simulink model "HANcoder_E407_GTSync_v4"  (R2018b)
settings: Solver=FixedStepDiscrete  StartTime=0.0  StopTime=1  FixedStep=0.01  RelTol=1e-3
PreLoadFcn:
  | librarySetup
  | eval([bdroot,'_startup']) %Calling [modelName]_startup.m
values from neighbouring files (symbols this model uses):
  basic_cycle_duration = TM12 + COMP_duration    (= 495)    [HANcoder_E407_GTSync_v4_startup.m]
  COM_Period = 100    [HANcoder_E407_GTSync_v4_startup.m]
  COM_Phase = COM_Period/2    (= 50)    [HANcoder_E407_GTSync_v4_startup.m]
  comm_delay_estimation = 20    [HANcoder_E407_GTSync_v4_startup.m]
  frequency_IRQ = 20    [HANcoder_E407_GTSync_v4_startup.m]
  HANtuneOverride = Simulink.Parameter    [HANcoder_E407_GTSync_v4_startup.m]
  idle_time_init = basic_cycle_duration*matrix_rows    (= 990)    [HANcoder_E407_GTSync_v4_startup.m]
  LED_ticks_toggle = 10000    [HANcoder_E407_GTSync_v4_startup.m]
  Master_Role = 1    [HANcoder_E407_GTSync_v4_startup.m]
  matrix_rows = 2    [HANcoder_E407_GTSync_v4_startup.m]
  Slave_Role = 2    [HANcoder_E407_GTSync_v4_startup.m]
  Sync_ID = 1    [HANcoder_E407_GTSync_v4_startup.m]
  time_difference_threshold = 500    [HANcoder_E407_GTSync_v4_startup.m]
  TM0 = basic_cycle_start    (= 5)    [HANcoder_E407_GTSync_v4_startup.m]
  TM1 = TM0 + COMM_duration    (= 105)    [HANcoder_E407_GTSync_v4_startup.m]
  TM10 = TM9  + COMP_duration    (= 465)    [HANcoder_E407_GTSync_v4_startup.m]
  TM11 = TM10 + COMP_duration    (= 475)    [HANcoder_E407_GTSync_v4_startup.m]
  TM12 = TM11 + COMP_duration    (= 485)    [HANcoder_E407_GTSync_v4_startup.m]
  TM2 = TM1 + COMP_duration    (= 115)    [HANcoder_E407_GTSync_v4_startup.m]
  TM3 = TM2 + COMP_duration    (= 125)    [HANcoder_E407_GTSync_v4_startup.m]
  TM4 = TM3 + COMM_duration    (= 225)    [HANcoder_E407_GTSync_v4_startup.m]
  TM5 = TM4 + COMP_duration    (= 235)    [HANcoder_E407_GTSync_v4_startup.m]
  TM6 = TM5 + COMM_duration    (= 335)    [HANcoder_E407_GTSync_v4_startup.m]
  TM7 = TM6 + COMP_duration    (= 345)    [HANcoder_E407_GTSync_v4_startup.m]
  TM8 = TM7 + COMM_duration    (= 445)    [HANcoder_E407_GTSync_v4_startup.m]
  TM9 = TM8  + COMP_duration    (= 455)    [HANcoder_E407_GTSync_v4_startup.m]
  Vote1_ID = 12    [HANcoder_E407_GTSync_v4_startup.m]
  Vote2_ID = 22    [HANcoder_E407_GTSync_v4_startup.m]
  Vote3_ID = 32    [HANcoder_E407_GTSync_v4_startup.m]
  wrap_up_threshold = basic_cycle_duration - time_difference_threshold*10    (= -4505)    [HANcoder_E407_GTSync_v4_startup.m]
undefined symbols (not defined in the file or in its folder): A0, A1, CON2
libraries: HANcoder_STM32_Target x22, simulink x3, hdlsllib x2, simulink_extras x1
(part 4 of 5)

== system HANcoder_E407_GTSync_v4/HANcoder STM32 Target - E407-STM32 algorithm/Global Ticks Increment/CAN Management/Matrix Cycle Manager/COMP Task - Vote Decision/Vote Decision ==
  note: Vote for lowest error count (lowest id wins at tie)
  note: Logic Analyzer - DEBUG
  note: Logic Analyzer - DEBUG
      | Start of COMP task
  Enable : EnablePort
  Cast : DataTypeConversion  OutDataTypeStr=uint8
  Constant : Constant
  Constant1 : Constant  Value=2
  Constant2 : Constant  Value=3
  Constant3 : Constant  OutDataTypeStr=boolean
  Constant4 : Constant
  Constant5 : Constant  Value=2
  Constant6 : Constant  Value=3
  Data Store Read : DataStoreRead  DataStoreName=sync_processed
  Data Store Read1 : DataStoreRead  DataStoreName=Board1_error_counter
  Data Store Read2 : DataStoreRead  DataStoreName=Board2_error_counter
  Data Store Read21 : DataStoreRead  DataStoreName=Master_ID
  Data Store Read3 : DataStoreRead  DataStoreName=Board3_error_counter
  Data Store Write3 : DataStoreWrite  DataStoreName=Toggle_Pin
  Data Store Write5 : DataStoreWrite  DataStoreName=Vote
  Ensure no self votes or failed master reelected : Subsystem
  Ensure no self votes or failed master reelected1 : Subsystem
  Ensure no self votes or failed master reelected2 : Subsystem
  Equal : RelationalOperator  Operator===  OutDataTypeStr=boolean  RndMeth=Simplest
  Equal5 : RelationalOperator  Operator===  OutDataTypeStr=boolean  RndMeth=Simplest
  Max : MinMax  Inputs=3
  Switch5 : Switch  Criteria=u2 > Threshold
  Switch6 : Switch  Criteria=u2 > Threshold
  Switch7 : Switch  Criteria=u2 > Threshold
  wires:
  Cast/1 -> Data Store Write5/1  "Vote_s"
  Equal/1 -> Switch6/2
  Data Store Read/1 -> Ensure no self votes or failed master reelected2/2(Sync Timeout), Ensure no self votes or failed master reelected1/2(Sync Timeout), Ensure no self votes or failed master reelected/2(Sync Timeout), Switch5/2
  Switch5/1 -> Cast/1
  Switch6/1 -> Switch5/3
  Data Store Read21/1 -> Switch5/1
  Ensure no self votes or failed master reelected2/1(Out1) -> Max/3
  Constant5/1 -> Switch7/1
  Ensure no self votes or failed master reelected1/1(Out1) -> Max/2, Equal5/2
  Constant4/1 -> Switch6/1
  Constant6/1 -> Switch7/3
  Switch7/1 -> Switch6/3
  Constant1/1 -> Ensure no self votes or failed master reelected1/1(Node ID)
  Constant2/1 -> Ensure no self votes or failed master reelected2/1(Node ID)
  Data Store Read1/1 -> Ensure no self votes or failed master reelected/3(Error counter)
  Equal5/1 -> Switch7/2
  Constant/1 -> Ensure no self votes or failed master reelected/1(Node ID)
  Max/1 -> Equal/2, Equal5/1
  Ensure no self votes or failed master reelected/1(Out1) -> Equal/1, Max/1
  Data Store Read2/1 -> Ensure no self votes or failed master reelected1/3(Error counter)
  Data Store Read3/1 -> Ensure no self votes or failed master reelected2/3(Error counter)
  Constant3/1 -> Data Store Write3/1

== system HANcoder_E407_GTSync_v4/HANcoder STM32 Target - E407-STM32 algorithm/Global Ticks Increment/CAN Management/Matrix Cycle Manager/COMP Task - Vote1 Count/Vote Count 1 ==
  note: Take vote into account if the board was synced
  note: Local Time Received Check
  note: Msg Received
  note: Logic Analyzer - DEBUG
      | Start of COMP task
  note: Logic Analyzer - DEBUG
  Msg Header : Inport
  Local Time Rx : Inport  Port=2
  Enable : EnablePort
  Abs : Abs
  Cast To Double : DataTypeConversion  OutDataTypeStr=double
  Cast To Double1 : DataTypeConversion  OutDataTypeStr=double
  Constant1 : Constant  OutDataTypeStr=boolean
  Constant3 : Constant  Value=Vote1_ID
  Constant4 : Constant  Value=time_difference_threshold
  Constant6 : Constant
  Data Store Read : DataStoreRead  DataStoreName=Board1_error_counter
  Data Store Read1 : DataStoreRead  DataStoreName=Local_Ticks
  Data Store Read5 : DataStoreRead  DataStoreName=Board1_error_counter
  Data Store Write : DataStoreWrite  DataStoreName=BC0_TM1_processed
  Data Store Write1 : DataStoreWrite  DataStoreName=Board1_error_counter
  Data Store Write2 : DataStoreWrite  DataStoreName=received_LT  DataStoreElements=received_LT.Local_Time_Board_1
  Data Store Write3 : DataStoreWrite  DataStoreName=Toggle_Pin
  Extra_Time : Subsystem
  GreaterThan : RelationalOperator  Operator=>  OutDataTypeStr=boolean  RndMeth=Simplest
  HIGH : Constant  OutDataTypeStr=boolean
  Minus : Sum  Inputs=+-
  NOT : Logic  Operator=NOT  IconShape=distinctive  AllPortsSameDT=off  OutDataTypeStr=boolean
  Plus : Sum
  RX-TX : Constant  Value=TM4-TM3  OutDataTypeStr=uint16
  Sum up new vote : Subsystem
  Switch2 : Switch  Criteria=u2 > Threshold
  Time_Difference_DEBUG : Subsystem
  wires:
  HIGH/1 -> Data Store Write/1
  Minus/1 -> Abs/1, Time_Difference_DEBUG/2(Time_Difference)
  Constant3/1 -> Time_Difference_DEBUG/1(RXID)
  Data Store Read1/1 -> Cast To Double1/1
  Abs/1 -> GreaterThan/1
  Constant4/1 -> GreaterThan/2
  Data Store Read5/1 -> Plus/1
  Plus/1 -> Switch2/1
  Constant6/1 -> Plus/2
  GreaterThan/1 -> Switch2/2, NOT/1
  Data Store Read/1 -> Switch2/3
  Switch2/1 -> Data Store Write1/1
  Extra_Time/1(Out1) -> Data Store Write2/1, Cast To Double/1
  Cast To Double1/1 -> Minus/2
  Msg Header/1 -> Sum up new vote/1(Msg Header)
  NOT/1 -> Sum up new vote/Enable
  Cast To Double/1 -> Minus/1
  RX-TX/1 -> Extra_Time/2(RX_Update_Delay)
  Local Time Rx/1 -> Extra_Time/1(Local_Time_RX)
  Constant1/1 -> Data Store Write3/1

== system HANcoder_E407_GTSync_v4/HANcoder STM32 Target - E407-STM32 algorithm/Global Ticks Increment/CAN Management/Matrix Cycle Manager/COMP Task - Vote2 Count/Vote Count 2 ==
  note: Msg Received
  note: Local Time Received Check
  note: Take vote into account if the board was synced
  note: Logic Analyzer - DEBUG
      | Start of COMP task
  note: Logic Analyzer - DEBUG
  Msg Header1 : Inport
  Local Time Rx : Inport  Port=2
  Enable : EnablePort
  Abs : Abs
  Cast To Double : DataTypeConversion  OutDataTypeStr=double
  Cast To Double1 : DataTypeConversion  OutDataTypeStr=double
  Constant1 : Constant  OutDataTypeStr=boolean
  Constant3 : Constant  Value=Vote2_ID
  Constant4 : Constant  Value=time_difference_threshold
  Constant6 : Constant
  Data Store Read : DataStoreRead  DataStoreName=Board2_error_counter
  Data Store Read1 : DataStoreRead  DataStoreName=Local_Ticks
  Data Store Read5 : DataStoreRead  DataStoreName=Board2_error_counter
  Data Store Write : DataStoreWrite  DataStoreName=BC0_TM2_processed
  Data Store Write1 : DataStoreWrite  DataStoreName=Board2_error_counter
  Data Store Write2 : DataStoreWrite  DataStoreName=received_LT  DataStoreElements=received_LT.Local_Time_Board_2
  Data Store Write3 : DataStoreWrite  DataStoreName=Toggle_Pin
  Extra_Time : Subsystem
  GreaterThan : RelationalOperator  Operator=>  OutDataTypeStr=boolean  RndMeth=Simplest
  HIGH : Constant  OutDataTypeStr=boolean
  Minus : Sum  Inputs=+-
  NOT : Logic  Operator=NOT  IconShape=distinctive  AllPortsSameDT=off  OutDataTypeStr=boolean
  Plus : Sum
  RX-TX : Constant  Value=TM6-TM5  OutDataTypeStr=uint16
  Sum up new vote : Subsystem
  Switch2 : Switch  Criteria=u2 > Threshold
  Time_Difference_DEBUG : Subsystem
  wires:
  Switch2/1 -> Data Store Write1/1
  Data Store Read/1 -> Switch2/3
  Constant6/1 -> Plus/2
  Plus/1 -> Switch2/1
  Data Store Read5/1 -> Plus/1
  Constant4/1 -> GreaterThan/2
  Abs/1 -> GreaterThan/1
  Data Store Read1/1 -> Cast To Double1/1
  Constant3/1 -> Time_Difference_DEBUG/1(RXID)
  Minus/1 -> Abs/1, Time_Difference_DEBUG/2(Time_Difference)
  HIGH/1 -> Data Store Write/1
  Cast To Double1/1 -> Minus/2
  GreaterThan/1 -> Switch2/2, NOT/1
  Msg Header1/1 -> Sum up new vote/1(Msg Header)
  NOT/1 -> Sum up new vote/Enable
  Cast To Double/1 -> Minus/1
  Extra_Time/1(Out1) -> Data Store Write2/1, Cast To Double/1
  RX-TX/1 -> Extra_Time/2(RX_Update_Delay)
  Local Time Rx/1 -> Extra_Time/1(Local_Time_RX)
  Constant1/1 -> Data Store Write3/1

== system HANcoder_E407_GTSync_v4/HANcoder STM32 Target - E407-STM32 algorithm/Global Ticks Increment/CAN Management/Matrix Cycle Manager/COMP Task - Vote3 Count/Vote Count 3 ==
  note: Local Time Received Check
  note: Msg Received
  note: Take vote into account if the board was synced
  note: Logic Analyzer - DEBUG
      | Start of COMP task
  note: Logic Analyzer - DEBUG
  Msg Header1 : Inport
  Local Time Rx : Inport  Port=2
  Enable : EnablePort
  Abs : Abs
  Cast To Double : DataTypeConversion  OutDataTypeStr=double
  Cast To Double1 : DataTypeConversion  OutDataTypeStr=double
  Constant1 : Constant  OutDataTypeStr=boolean
  Constant3 : Constant  Value=Vote3_ID
  Constant4 : Constant  Value=time_difference_threshold
  Constant6 : Constant
  Data Store Read : DataStoreRead  DataStoreName=Board3_error_counter
  Data Store Read1 : DataStoreRead  DataStoreName=Local_Ticks
  Data Store Read5 : DataStoreRead  DataStoreName=Board3_error_counter
  Data Store Write : DataStoreWrite  DataStoreName=BC0_TM3_processed
  Data Store Write1 : DataStoreWrite  DataStoreName=Board3_error_counter
  Data Store Write2 : DataStoreWrite  DataStoreName=received_LT  DataStoreElements=received_LT.Local_Time_Board_3
  Data Store Write3 : DataStoreWrite  DataStoreName=Toggle_Pin
  Extra_Time : Subsystem
  GreaterThan : RelationalOperator  Operator=>  OutDataTypeStr=boolean  RndMeth=Simplest
  HIGH : Constant  OutDataTypeStr=boolean
  Minus : Sum  Inputs=+-
  NOT : Logic  Operator=NOT  IconShape=distinctive  AllPortsSameDT=off  OutDataTypeStr=boolean
  Plus : Sum
  RX-TX : Constant  Value=TM8-TM7  OutDataTypeStr=uint16
  Sum up new vote : Subsystem
  Switch2 : Switch  Criteria=u2 > Threshold
  Time_Difference_DEBUG : Subsystem
  wires:
  HIGH/1 -> Data Store Write/1
  Minus/1 -> Time_Difference_DEBUG/2(Time_Difference), Abs/1
  Constant3/1 -> Time_Difference_DEBUG/1(RXID)
  Data Store Read1/1 -> Cast To Double1/1
  Abs/1 -> GreaterThan/1
  Constant4/1 -> GreaterThan/2
  Data Store Read5/1 -> Plus/1
  Plus/1 -> Switch2/1
  Constant6/1 -> Plus/2
  Data Store Read/1 -> Switch2/3
  Switch2/1 -> Data Store Write1/1
  Cast To Double1/1 -> Minus/2
  GreaterThan/1 -> NOT/1, Switch2/2
  Msg Header1/1 -> Sum up new vote/1(Msg Header)
  NOT/1 -> Sum up new vote/Enable
  Cast To Double/1 -> Minus/1
  Extra_Time/1(Out1) -> Data Store Write2/1, Cast To Double/1
  RX-TX/1 -> Extra_Time/2(RX_Update_Delay)
  Local Time Rx/1 -> Extra_Time/1(Local_Time_RX)
  Constant1/1 -> Data Store Write3/1

== system HANcoder_E407_GTSync_v4/HANcoder STM32 Target - E407-STM32 algorithm/Global Ticks Increment/CAN Recieve/RxID_CAN/Sync_ID_CAN/CAN receive ==
  In1 : Inport
  Enabled Subsystem : Subsystem  TreatAsAtomicUnit=on
  S-Function : M-S-Function  FunctionName=sfcn_can_receive  Parameters=tsamp, canBus, outputNumber, dataType, byteOrder
  Out1 : Outport
  Out2 : Outport  Port=2
  Out3 : Outport  Port=3
  Out4 : Outport  Port=4
  Out5 : Outport  Port=5
  Out6 : Outport  Port=6
  Out7 : Outport  Port=7
  Out8 : Outport  Port=8
  Out9 : Outport  Port=9
  wires:
  S-Function/9 -> Enabled Subsystem/8(In8)
  S-Function/4 -> Enabled Subsystem/3(In3)
  S-Function/5 -> Enabled Subsystem/4(In4)
  S-Function/8 -> Enabled Subsystem/7(In7)
  S-Function/7 -> Enabled Subsystem/6(In6)
  S-Function/6 -> Enabled Subsystem/5(In5)
  Enabled Subsystem/8(Out8) -> Out9/1
  Enabled Subsystem/7(Out7) -> Out8/1
  Enabled Subsystem/6(Out6) -> Out7/1
  Enabled Subsystem/5(Out5) -> Out6/1
  Enabled Subsystem/4(Out4) -> Out5/1
  Enabled Subsystem/3(Out3) -> Out4/1
  Enabled Subsystem/2(Out2) -> Out3/1
  Enabled Subsystem/1(Out1) -> Out2/1
  S-Function/3 -> Enabled Subsystem/2(In2)
  S-Function/2 -> Enabled Subsystem/1(In1)
  S-Function/1 -> Out1/1, Enabled Subsystem/Enable
  In1/1 -> S-Function/1

== system HANcoder_E407_GTSync_v4/HANcoder STM32 Target - E407-STM32 algorithm/Global Ticks Increment/CAN Recieve/RxID_CAN/Vote1_ID_CAN/CAN receive ==
  In1 : Inport
  Enabled Subsystem : Subsystem  TreatAsAtomicUnit=on
  S-Function : M-S-Function  FunctionName=sfcn_can_receive  Parameters=tsamp, canBus, outputNumber, dataType, byteOrder
  Out1 : Outport
  Out2 : Outport  Port=2
  Out3 : Outport  Port=3
  Out4 : Outport  Port=4
  Out5 : Outport  Port=5
  Out6 : Outport  Port=6
  Out7 : Outport  Port=7
  Out8 : Outport  Port=8
  Out9 : Outport  Port=9
  wires:
  In1/1 -> S-Function/1
  S-Function/1 -> Enabled Subsystem/Enable, Out1/1
  S-Function/2 -> Enabled Subsystem/1(In1)
  S-Function/3 -> Enabled Subsystem/2(In2)
  Enabled Subsystem/1(Out1) -> Out2/1
  Enabled Subsystem/2(Out2) -> Out3/1
  Enabled Subsystem/3(Out3) -> Out4/1
  Enabled Subsystem/4(Out4) -> Out5/1
  Enabled Subsystem/5(Out5) -> Out6/1
  Enabled Subsystem/6(Out6) -> Out7/1
  Enabled Subsystem/7(Out7) -> Out8/1
  Enabled Subsystem/8(Out8) -> Out9/1
  S-Function/6 -> Enabled Subsystem/5(In5)
  S-Function/7 -> Enabled Subsystem/6(In6)
  S-Function/8 -> Enabled Subsystem/7(In7)
  S-Function/5 -> Enabled Subsystem/4(In4)
  S-Function/4 -> Enabled Subsystem/3(In3)
  S-Function/9 -> Enabled Subsystem/8(In8)

== system HANcoder_E407_GTSync_v4/HANcoder STM32 Target - E407-STM32 algorithm/Global Ticks Increment/CAN Recieve/RxID_CAN/Vote2_ID_CAN/CAN receive ==
  In1 : Inport
  Enabled Subsystem : Subsystem  TreatAsAtomicUnit=on
  S-Function : M-S-Function  FunctionName=sfcn_can_receive  Parameters=tsamp, canBus, outputNumber, dataType, byteOrder
  Out1 : Outport
  Out2 : Outport  Port=2
  Out3 : Outport  Port=3
  Out4 : Outport  Port=4
  Out5 : Outport  Port=5
  Out6 : Outport  Port=6
  Out7 : Outport  Port=7
  Out8 : Outport  Port=8
  Out9 : Outport  Port=9
  wires:
  S-Function/9 -> Enabled Subsystem/8(In8)
  S-Function/4 -> Enabled Subsystem/3(In3)
  S-Function/5 -> Enabled Subsystem/4(In4)
  S-Function/8 -> Enabled Subsystem/7(In7)
  S-Function/7 -> Enabled Subsystem/6(In6)
  S-Function/6 -> Enabled Subsystem/5(In5)
  Enabled Subsystem/8(Out8) -> Out9/1
  Enabled Subsystem/7(Out7) -> Out8/1
  Enabled Subsystem/6(Out6) -> Out7/1
  Enabled Subsystem/5(Out5) -> Out6/1
  Enabled Subsystem/4(Out4) -> Out5/1
  Enabled Subsystem/3(Out3) -> Out4/1
  Enabled Subsystem/2(Out2) -> Out3/1
  Enabled Subsystem/1(Out1) -> Out2/1
  S-Function/3 -> Enabled Subsystem/2(In2)
  S-Function/2 -> Enabled Subsystem/1(In1)
  S-Function/1 -> Out1/1, Enabled Subsystem/Enable
  In1/1 -> S-Function/1

== system HANcoder_E407_GTSync_v4/HANcoder STM32 Target - E407-STM32 algorithm/Global Ticks Increment/CAN Recieve/RxID_CAN/Vote3_ID_CAN/CAN receive ==
  In1 : Inport
  Enabled Subsystem : Subsystem  TreatAsAtomicUnit=on
  S-Function : M-S-Function  FunctionName=sfcn_can_receive  Parameters=tsamp, canBus, outputNumber, dataType, byteOrder
  Out1 : Outport
  Out2 : Outport  Port=2
  Out3 : Outport  Port=3
  Out4 : Outport  Port=4
  Out5 : Outport  Port=5
  Out6 : Outport  Port=6
  Out7 : Outport  Port=7
  Out8 : Outport  Port=8
  Out9 : Outport  Port=9
  wires:
  In1/1 -> S-Function/1
  S-Function/1 -> Enabled Subsystem/Enable, Out1/1
  S-Function/2 -> Enabled Subsystem/1(In1)
  S-Function/3 -> Enabled Subsystem/2(In2)
  Enabled Subsystem/1(Out1) -> Out2/1
  Enabled Subsystem/2(Out2) -> Out3/1
  Enabled Subsystem/3(Out3) -> Out4/1
  Enabled Subsystem/4(Out4) -> Out5/1
  Enabled Subsystem/5(Out5) -> Out6/1
  Enabled Subsystem/6(Out6) -> Out7/1
  Enabled Subsystem/7(Out7) -> Out8/1
  Enabled Subsystem/8(Out8) -> Out9/1
  S-Function/6 -> Enabled Subsystem/5(In5)
  S-Function/7 -> Enabled Subsystem/6(In6)
  S-Function/8 -> Enabled Subsystem/7(In7)
  S-Function/5 -> Enabled Subsystem/4(In4)
  S-Function/4 -> Enabled Subsystem/3(In3)
  S-Function/9 -> Enabled Subsystem/8(In8)

== system HANcoder_E407_GTSync_v4/HANcoder STM32 Target - E407-STM32 algorithm/Global Ticks Increment/CAN Management/Matrix Cycle Manager/COMP Task - Check Timeouts/Timeout and Board error counter/Timeout Counter 1 DEBUG ==
  Timeout : Inport
  Constant : Constant
  Data Store Memory : DataStoreMemory  DataStoreName=BC0_TM1_timeout_counter  ReadBeforeWriteMsg=warning  WriteAfterWriteMsg=warning  WriteAfterReadMsg=warning  ShowAdditionalParam=off
  Data Store Read : DataStoreRead  DataStoreName=BC0_TM1_timeout_counter
  Data Store Read1 : DataStoreRead  DataStoreName=BC0_TM1_timeout_counter
  Data Store Write : DataStoreWrite  DataStoreName=BC0_TM1_timeout_counter
  Plus : Sum
  Switch : Switch  Criteria=u2 > Threshold
  wires:
  Timeout/1 -> Switch/2
  Switch/1 -> Data Store Write/1  "TM1_timeout_counter_s"
  Data Store Read1/1 -> Plus/1
  Constant/1 -> Plus/2
  Plus/1 -> Switch/1
  Data Store Read/1 -> Switch/3

== system HANcoder_E407_GTSync_v4/HANcoder STM32 Target - E407-STM32 algorithm/Global Ticks Increment/CAN Management/Matrix Cycle Manager/COMP Task - Check Timeouts/Timeout and Board error counter/Timeout Counter 2 DEBUG ==
  Timeout : Inport
  Constant : Constant
  Data Store Memory : DataStoreMemory  DataStoreName=BC0_TM2_timeout_counter  ReadBeforeWriteMsg=warning  WriteAfterWriteMsg=warning  WriteAfterReadMsg=warning  ShowAdditionalParam=off
  Data Store Read : DataStoreRead  DataStoreName=BC0_TM2_timeout_counter
  Data Store Read1 : DataStoreRead  DataStoreName=BC0_TM2_timeout_counter
  Data Store Write : DataStoreWrite  DataStoreName=BC0_TM2_timeout_counter
  Plus : Sum
  Switch : Switch  Criteria=u2 > Threshold
  wires:
  Data Store Read/1 -> Switch/3
  Plus/1 -> Switch/1
  Constant/1 -> Plus/2
  Data Store Read1/1 -> Plus/1
  Switch/1 -> Data Store Write/1  "TM2_timeout_counter_s"
  Timeout/1 -> Switch/2

== system HANcoder_E407_GTSync_v4/HANcoder STM32 Target - E407-STM32 algorithm/Global Ticks Increment/CAN Management/Matrix Cycle Manager/COMP Task - Check Timeouts/Timeout and Board error counter/Timeout Counter 3 DEBUG ==
  Timeout : Inport
  Constant : Constant
  Data Store Memory : DataStoreMemory  DataStoreName=BC0_TM3_timeout_counter  ReadBeforeWriteMsg=warning  WriteAfterWriteMsg=warning  WriteAfterReadMsg=warning  ShowAdditionalParam=off
  Data Store Read : DataStoreRead  DataStoreName=BC0_TM3_timeout_counter
  Data Store Read1 : DataStoreRead  DataStoreName=BC0_TM3_timeout_counter
  Data Store Write : DataStoreWrite  DataStoreName=BC0_TM3_timeout_counter
  Plus : Sum
  Switch : Switch  Criteria=u2 > Threshold
  wires:
  Timeout/1 -> Switch/2
  Switch/1 -> Data Store Write/1  "TM3_timeout_counter_s"
  Data Store Read1/1 -> Plus/1
  Constant/1 -> Plus/2
  Plus/1 -> Switch/1
  Data Store Read/1 -> Switch/3

== system HANcoder_E407_GTSync_v4/HANcoder STM32 Target - E407-STM32 algorithm/Global Ticks Increment/CAN Management/Matrix Cycle Manager/COMP Task - New Master/New Master/Votes recount to choose Master ==
  note: If no votes received: RESET Board
  note: Add self node vote
  Compare To Constant : simulink/Logic and Bit Operations/Compare To Constant  relop===  const=0  OutDataTypeStr=boolean
  Constant : Constant  Value=0
  Constant15 : Constant
  Constant16 : Constant  Value=2
  Constant17 : Constant  Value=3
  Data Store Read25 : DataStoreRead  DataStoreName=votes  DataStoreElements=votes.First_Board#votes.Second_Board#votes.Third_Board
  Data Store Read29 : DataStoreRead  DataStoreName=Vote
  Equal{,17..19} (4 alike) : RelationalOperator  Operator===  OutDataTypeStr=boolean  RndMeth=Simplest
  Find Nonzero Elements : Find  NumberOfInputDimensions=3  IndexMode=Zero-based  OutDataTypeStr=int32
  Index Corrector : Constant
  Max : MinMax  Function=max
  Max1 : MinMax  Function=max
  Min : MinMax
  Minus : Sum
  Mux : Mux  Inputs=3
  Mux1 : Mux  Inputs=3
  Plus : Sum
  Plus1 : Sum
  Plus2 : Sum
  Subtract : Sum  Inputs=+-
  Master_ID_s : Outport
  Reset Board : Outport  Port=2
  wires:
  Data Store Read25/1 -> Plus/1, Mux1/1
  Equal18/1 -> Plus1/2
  Plus/1 -> Mux/1
  Constant15/1 -> Equal17/1
  Plus1/1 -> Mux/2
  Min/1 -> Minus/1
  Index Corrector/1 -> Minus/2
  Data Store Read25/2 -> Plus1/1, Mux1/2
  Plus2/1 -> Mux/3
  Equal19/1 -> Plus2/2
  Data Store Read29/1 -> Equal19/2, Equal18/2, Equal17/2
  Find Nonzero Elements/1 -> Min/1
  Equal17/1 -> Plus/2
  Subtract/1 -> Compare To Constant/1
  Constant16/1 -> Equal18/1
  Max/1 -> Subtract/2
  Mux/1 -> Subtract/1, Max/1
  Data Store Read25/3 -> Plus2/1, Mux1/3
  Constant17/1 -> Equal19/1
  Compare To Constant/1 -> Find Nonzero Elements/1
  Minus/1 -> Master_ID_s/1  "Master_ID_s"
  Mux1/1 -> Max1/1
  Max1/1 -> Equal/2
  Constant/1 -> Equal/1
  Equal/1 -> Reset Board/1

== system HANcoder_E407_GTSync_v4/HANcoder STM32 Target - E407-STM32 algorithm/Global Ticks Increment/CAN Management/Matrix Cycle Manager/COMP Task - Update LT/Local Time Update/Extra_Time ==
  note: Desync
      | Time from actual Rx until
      | expected Rx time
  note: Time from expected Rx
      | until new TM
  Local_Time_RX : Inport
  " " : Constant  Value=COM_Phase  OutDataTypeStr=uint16
  Constant : Constant  Value=TM0  OutDataTypeStr=uint16
  Data Store Read : DataStoreRead  DataStoreName=Msg_Rx_Ticks
  Minus : Sum  Inputs=+++
  Minus1 : Sum  Inputs=+-
  Minus2 : Sum  Inputs=++-
  Task_phase : Constant  Value=COM_Phase  OutDataTypeStr=uint16
  Task_time : Constant  Value=TM1-TM0  OutDataTypeStr=uint16
  Out1 : Outport  OutDataTypeStr=uint16
  wires:
  Local_Time_RX/1 -> Minus/1
  Minus/1 -> Out1/1
  Minus2/1 -> Minus/2
  Minus1/1 -> Minus/3
  Task_phase/1 -> Minus1/2
  Task_time/1 -> Minus1/1
  Constant/1 -> Minus2/1
  " "/1 -> Minus2/2
  Data Store Read/1 -> Minus2/3

== system HANcoder_E407_GTSync_v4/HANcoder STM32 Target - E407-STM32 algorithm/Global Ticks Increment/CAN Management/Matrix Cycle Manager/COMP Task - Update LT/Local Time Update/Process Time Difference ==
  Rx_Time : Inport
  Local_Time : Inport  Port=2
  Check_Wrap_up : Subsystem
  Check_Wrap_up1 : Subsystem
  Minus : Sum  Inputs=+-
  Time_Difference : Outport
  wires:
  Minus/1 -> Time_Difference/1
  Rx_Time/1 -> Check_Wrap_up/1(In1)
  Local_Time/1 -> Check_Wrap_up1/1(In1)
  Check_Wrap_up/1(Out1) -> Minus/1
  Check_Wrap_up1/1(Out1) -> Minus/2

== system HANcoder_E407_GTSync_v4/HANcoder STM32 Target - E407-STM32 algorithm/Global Ticks Increment/CAN Management/Matrix Cycle Manager/COMP Task - Update LT/Local Time Update/Time_Difference_DEBUG ==
  RXID : Inport
  Time_Difference : Inport  Port=2
  Constant : Constant  Value=Vote1_ID
  Constant1 : Constant  Value=Vote2_ID
  Constant2 : Constant  Value=Vote3_ID
  Constant3 : Constant  Value=Sync_ID
  Data Store Read : DataStoreRead  DataStoreName=time_difference_sync
  Data Store Read1 : DataStoreRead  DataStoreName=time_difference_vote1
  Data Store Read2 : DataStoreRead  DataStoreName=time_difference_vote2
  Data Store Read3 : DataStoreRead  DataStoreName=time_difference_vote3
  Data Store Write : DataStoreWrite  DataStoreName=time_difference_sync
  Data Store Write1 : DataStoreWrite  DataStoreName=time_difference_vote1
  Data Store Write2 : DataStoreWrite  DataStoreName=time_difference_vote2
  Data Store Write3 : DataStoreWrite  DataStoreName=time_difference_vote3
  Equal{,1..3} (4 alike) : RelationalOperator  Operator===  OutDataTypeStr=boolean  RndMeth=Simplest
  Switch{,1..3} (4 alike) : Switch  Criteria=u2 > Threshold
  wires:
  Time_Difference/1 -> Switch/1, Switch1/1, Switch2/1, Switch3/1
  Constant3/1 -> Equal/1
  Constant/1 -> Equal1/1
  Constant1/1 -> Equal2/1
  Constant2/1 -> Equal3/1
  RXID/1 -> Equal3/2, Equal2/2, Equal1/2, Equal/2
  Equal/1 -> Switch/2
  Equal1/1 -> Switch1/2
  Equal2/1 -> Switch2/2
  Switch/1 -> Data Store Write/1  "bc1_time_difference_sync_s"
  Switch1/1 -> Data Store Write1/1  "bc1_time_difference_vote1_s"
  Switch2/1 -> Data Store Write2/1  "bc1_time_difference_vote2_s"
  Equal3/1 -> Switch3/2
  Switch3/1 -> Data Store Write3/1  "bc1_time_difference_vote3_s"
  Data Store Read/1 -> Switch/3
  Data Store Read1/1 -> Switch1/3
  Data Store Read2/1 -> Switch2/3
  Data Store Read3/1 -> Switch3/3

== system HANcoder_E407_GTSync_v4/HANcoder STM32 Target - E407-STM32 algorithm/Global Ticks Increment/CAN Management/Matrix Cycle Manager/COMP Task - Update LT1/Local Time Update/Extra_Time ==
  Local_Time_RX : Inport
  RX_Update_Delay : Inport  Port=2
  Constant : Constant  Value=COM_Phase  OutDataTypeStr=uint16
  Minus : Sum  Inputs=++-
  Out1 : Outport  OutDataTypeStr=uint16
  wires:
  Local_Time_RX/1 -> Minus/1
  Minus/1 -> Out1/1
  RX_Update_Delay/1 -> Minus/2
  Constant/1 -> Minus/3

== system HANcoder_E407_GTSync_v4/HANcoder STM32 Target - E407-STM32 algorithm/Global Ticks Increment/CAN Management/Matrix Cycle Manager/COMP Task - Update LT1/Local Time Update/Process Time Difference ==
  Rx_Time : Inport
  Local_Time : Inport  Port=2
  Check_Wrap_up : Subsystem
  Check_Wrap_up1 : Subsystem
  Minus : Sum  Inputs=+-
  Time_Difference : Outport
  wires:
  Check_Wrap_up1/1(Out1) -> Minus/2
  Check_Wrap_up/1(Out1) -> Minus/1
  Local_Time/1 -> Check_Wrap_up1/1(In1)
  Rx_Time/1 -> Check_Wrap_up/1(In1)
  Minus/1 -> Time_Difference/1

== system HANcoder_E407_GTSync_v4/HANcoder STM32 Target - E407-STM32 algorithm/Global Ticks Increment/CAN Management/Matrix Cycle Manager/COMP Task - Update LT1/Local Time Update/Time_Difference_DEBUG ==
  RXID : Inport
  Time_Difference : Inport  Port=2
  Constant : Constant  Value=Vote1_ID
  Constant1 : Constant  Value=Vote2_ID
  Constant2 : Constant  Value=Vote3_ID
  Constant3 : Constant  Value=Sync_ID
  Data Store Read : DataStoreRead  DataStoreName=time_difference_sync
  Data Store Read1 : DataStoreRead  DataStoreName=time_difference_vote1
  Data Store Read2 : DataStoreRead  DataStoreName=time_difference_vote2
  Data Store Read3 : DataStoreRead  DataStoreName=time_difference_vote3
  Data Store Write : DataStoreWrite  DataStoreName=time_difference_sync
  Data Store Write1 : DataStoreWrite  DataStoreName=time_difference_vote1
  Data Store Write2 : DataStoreWrite  DataStoreName=time_difference_vote2
  Data Store Write3 : DataStoreWrite  DataStoreName=time_difference_vote3
  Equal{,1..3} (4 alike) : RelationalOperator  Operator===  OutDataTypeStr=boolean  RndMeth=Simplest
  Switch{,1..3} (4 alike) : Switch  Criteria=u2 > Threshold
  wires:
  Data Store Read3/1 -> Switch3/3
  Data Store Read2/1 -> Switch2/3
  Data Store Read1/1 -> Switch1/3
  Data Store Read/1 -> Switch/3
  Switch3/1 -> Data Store Write3/1  "time_difference_vote3_s"
  Equal3/1 -> Switch3/2
  Switch2/1 -> Data Store Write2/1  "time_difference_vote2_s"
  Switch1/1 -> Data Store Write1/1  "time_difference_vote1_s"
  Switch/1 -> Data Store Write/1  "time_difference_sync_s"
  Equal2/1 -> Switch2/2
  Equal1/1 -> Switch1/2
  Equal/1 -> Switch/2
  RXID/1 -> Equal/2, Equal1/2, Equal2/2, Equal3/2
  Constant2/1 -> Equal3/1
  Constant1/1 -> Equal2/1
  Constant/1 -> Equal1/1
  Constant3/1 -> Equal/1
  Time_Difference/1 -> Switch3/1, Switch2/1, Switch1/1, Switch/1

== system HANcoder_E407_GTSync_v4/HANcoder STM32 Target - E407-STM32 algorithm/Global Ticks Increment/CAN Management/Matrix Cycle Manager/COMP Task - Vote Decision/Vote Decision/Ensure no self votes or failed master reelected ==
  Node ID : Inport
  Sync Timeout : Inport  Port=2
  Error counter : Inport  Port=3
  AND : Logic  IconShape=distinctive  AllPortsSameDT=off  OutDataTypeStr=boolean
  Data Store Read : DataStoreRead  DataStoreName=Board_ID
  Data Store Read2 : DataStoreRead  DataStoreName=Master_ID
  Equal1 : RelationalOperator  Operator===  OutDataTypeStr=boolean  RndMeth=Simplest
  Equal2 : RelationalOperator  Operator===  OutDataTypeStr=boolean  RndMeth=Simplest
  MAX error count : Constant  Value=4294967295  OutDataTypeStr=uint32
  NOT : Logic  Operator=NOT  IconShape=distinctive  AllPortsSameDT=off  OutDataTypeStr=boolean
  OR : Logic  Operator=OR  IconShape=distinctive  AllPortsSameDT=off  OutDataTypeStr=boolean
  Switch : Switch  Criteria=u2 > Threshold
  Out1 : Outport
  wires:
  Equal1/1 -> OR/1
  Data Store Read/1 -> Equal1/2
  MAX error count/1 -> Switch/1
  Switch/1 -> Out1/1
  Error counter/1 -> Switch/3
  Node ID/1 -> Equal1/1, Equal2/2
  Sync Timeout/1 -> NOT/1
  Data Store Read2/1 -> Equal2/1
  Equal2/1 -> AND/1
  NOT/1 -> AND/2
  AND/1 -> OR/2
  OR/1 -> Switch/2

== system HANcoder_E407_GTSync_v4/HANcoder STM32 Target - E407-STM32 algorithm/Global Ticks Increment/CAN Management/Matrix Cycle Manager/COMP Task - Vote Decision/Vote Decision/Ensure no self votes or failed master reelected1 ==
  Node ID : Inport
  Sync Timeout : Inport  Port=2
  Error counter : Inport  Port=3
  AND : Logic  IconShape=distinctive  AllPortsSameDT=off  OutDataTypeStr=boolean
  Data Store Read : DataStoreRead  DataStoreName=Board_ID
  Data Store Read2 : DataStoreRead  DataStoreName=Master_ID
  Equal1 : RelationalOperator  Operator===  OutDataTypeStr=boolean  RndMeth=Simplest
  Equal2 : RelationalOperator  Operator===  OutDataTypeStr=boolean  RndMeth=Simplest
  MAX error count : Constant  Value=4294967295  OutDataTypeStr=uint32
  NOT : Logic  Operator=NOT  IconShape=distinctive  AllPortsSameDT=off  OutDataTypeStr=boolean
  OR : Logic  Operator=OR  IconShape=distinctive  AllPortsSameDT=off  OutDataTypeStr=boolean
  Switch : Switch  Criteria=u2 > Threshold
  Out1 : Outport
  wires:
  OR/1 -> Switch/2
  AND/1 -> OR/2
  NOT/1 -> AND/2
  Equal2/1 -> AND/1
  Data Store Read2/1 -> Equal2/1
  Sync Timeout/1 -> NOT/1
  Node ID/1 -> Equal2/2, Equal1/1
  Error counter/1 -> Switch/3
  Switch/1 -> Out1/1
  MAX error count/1 -> Switch/1
  Data Store Read/1 -> Equal1/2
  Equal1/1 -> OR/1

== system HANcoder_E407_GTSync_v4/HANcoder STM32 Target - E407-STM32 algorithm/Global Ticks Increment/CAN Management/Matrix Cycle Manager/COMP Task - Vote Decision/Vote Decision/Ensure no self votes or failed master reelected2 ==
  Node ID : Inport
  Sync Timeout : Inport  Port=2
  Error counter : Inport  Port=3
  AND : Logic  IconShape=distinctive  AllPortsSameDT=off  OutDataTypeStr=boolean
  Data Store Read : DataStoreRead  DataStoreName=Board_ID
  Data Store Read2 : DataStoreRead  DataStoreName=Master_ID
  Equal1 : RelationalOperator  Operator===  OutDataTypeStr=boolean  RndMeth=Simplest
  Equal2 : RelationalOperator  Operator===  OutDataTypeStr=boolean  RndMeth=Simplest
  MAX error count : Constant  Value=4294967295  OutDataTypeStr=uint32
  NOT : Logic  Operator=NOT  IconShape=distinctive  AllPortsSameDT=off  OutDataTypeStr=boolean
  OR : Logic  Operator=OR  IconShape=distinctive  AllPortsSameDT=off  OutDataTypeStr=boolean
  Switch : Switch  Criteria=u2 > Threshold
  Out1 : Outport
  wires:
  Equal1/1 -> OR/1
  Data Store Read/1 -> Equal1/2
  MAX error count/1 -> Switch/1
  Switch/1 -> Out1/1
  Error counter/1 -> Switch/3
  Node ID/1 -> Equal1/1, Equal2/2
  Sync Timeout/1 -> NOT/1
  Data Store Read2/1 -> Equal2/1
  Equal2/1 -> AND/1
  NOT/1 -> AND/2
  AND/1 -> OR/2
  OR/1 -> Switch/2

== system HANcoder_E407_GTSync_v4/HANcoder STM32 Target - E407-STM32 algorithm/Global Ticks Increment/CAN Management/Matrix Cycle Manager/COMP Task - Vote1 Count/Vote Count 1/Extra_Time ==
  Local_Time_RX : Inport
  RX_Update_Delay : Inport  Port=2
  Constant : Constant  Value=COM_Phase  OutDataTypeStr=uint16
  Minus : Sum  Inputs=++-
  Out1 : Outport  OutDataTypeStr=uint16
  wires:
  Local_Time_RX/1 -> Minus/1
  Minus/1 -> Out1/1
  RX_Update_Delay/1 -> Minus/2
  Constant/1 -> Minus/3

== system HANcoder_E407_GTSync_v4/HANcoder STM32 Target - E407-STM32 algorithm/Global Ticks Increment/CAN Management/Matrix Cycle Manager/COMP Task - Vote1 Count/Vote Count 1/Sum up new vote ==
  note: Registering votes
  Msg Header : Inport
  Enable : EnablePort
  Add : Sum
  Add1 : Sum
  Add2 : Sum
  Constant10 : Constant
  Constant11 : Constant  Value=2
  Constant12 : Constant  Value=3
  Data Store Read15 : DataStoreRead  DataStoreName=votes  DataStoreElements=votes.First_Board
  Data Store Read16 : DataStoreRead  DataStoreName=votes  DataStoreElements=votes.Second_Board
  Data Store Read17 : DataStoreRead  DataStoreName=votes  DataStoreElements=votes.Third_Board
  Data Store Write12 : DataStoreWrite  DataStoreName=votes  DataStoreElements=votes.First_Board#votes.Second_Board#votes.Third_Board
  Equal13 : RelationalOperator  Operator===  OutDataTypeStr=boolean  RndMeth=Simplest
  Equal15 : RelationalOperator  Operator===  OutDataTypeStr=boolean  RndMeth=Simplest
  Equal17 : RelationalOperator  Operator===  OutDataTypeStr=boolean  RndMeth=Simplest
  wires:
  Equal17/1 -> Add2/2
  Constant12/1 -> Equal17/1
  Add2/1 -> Data Store Write12/3
  Msg Header/1 -> Equal17/2, Equal15/2, Equal13/2
  Constant11/1 -> Equal15/1
  Data Store Read16/1 -> Add1/1
  Data Store Read15/1 -> Add/1
  Equal15/1 -> Add1/2
  Data Store Read17/1 -> Add2/1
  Constant10/1 -> Equal13/1
  Add1/1 -> Data Store Write12/2
  Add/1 -> Data Store Write12/1
  Equal13/1 -> Add/2

== system HANcoder_E407_GTSync_v4/HANcoder STM32 Target - E407-STM32 algorithm/Global Ticks Increment/CAN Management/Matrix Cycle Manager/COMP Task - Vote1 Count/Vote Count 1/Time_Difference_DEBUG ==
  RXID : Inport
  Time_Difference : Inport  Port=2
  Constant : Constant  Value=Vote1_ID
  Constant1 : Constant  Value=Vote2_ID
  Constant2 : Constant  Value=Vote3_ID
  Constant3 : Constant  Value=Sync_ID
  Data Store Read : DataStoreRead  DataStoreName=time_difference_sync
  Data Store Read1 : DataStoreRead  DataStoreName=time_difference_vote1
  Data Store Read2 : DataStoreRead  DataStoreName=time_difference_vote2
  Data Store Read3 : DataStoreRead  DataStoreName=time_difference_vote3
  Data Store Write : DataStoreWrite  DataStoreName=time_difference_sync
  Data Store Write1 : DataStoreWrite  DataStoreName=time_difference_vote1
  Data Store Write2 : DataStoreWrite  DataStoreName=time_difference_vote2
  Data Store Write3 : DataStoreWrite  DataStoreName=time_difference_vote3
  Equal{,1..3} (4 alike) : RelationalOperator  Operator===  OutDataTypeStr=boolean  RndMeth=Simplest
  Switch{,1..3} (4 alike) : Switch  Criteria=u2 > Threshold
  wires:
  Time_Difference/1 -> Switch/1, Switch1/1, Switch2/1, Switch3/1
  Constant3/1 -> Equal/1
  Constant/1 -> Equal1/1
  Constant1/1 -> Equal2/1
  Constant2/1 -> Equal3/1
  RXID/1 -> Equal3/2, Equal2/2, Equal1/2, Equal/2
  Equal/1 -> Switch/2
  Equal1/1 -> Switch1/2
  Equal2/1 -> Switch2/2
  Switch/1 -> Data Store Write/1  "time_difference_sync_s1"
  Switch1/1 -> Data Store Write1/1  "time_difference_vote1_s1"
  Switch2/1 -> Data Store Write2/1  "time_difference_vote2_s1"
  Equal3/1 -> Switch3/2
  Switch3/1 -> Data Store Write3/1  "time_difference_vote3_s1"
  Data Store Read/1 -> Switch/3
  Data Store Read1/1 -> Switch1/3
  Data Store Read2/1 -> Switch2/3
  Data Store Read3/1 -> Switch3/3

== system HANcoder_E407_GTSync_v4/HANcoder STM32 Target - E407-STM32 algorithm/Global Ticks Increment/CAN Management/Matrix Cycle Manager/COMP Task - Vote2 Count/Vote Count 2/Extra_Time ==
  Local_Time_RX : Inport
  RX_Update_Delay : Inport  Port=2
  Constant : Constant  Value=COM_Phase  OutDataTypeStr=uint16
  Minus : Sum  Inputs=++-
  Out1 : Outport  OutDataTypeStr=uint16
  wires:
  Local_Time_RX/1 -> Minus/1
  Minus/1 -> Out1/1
  RX_Update_Delay/1 -> Minus/2
  Constant/1 -> Minus/3

== system HANcoder_E407_GTSync_v4/HANcoder STM32 Target - E407-STM32 algorithm/Global Ticks Increment/CAN Management/Matrix Cycle Manager/COMP Task - Vote2 Count/Vote Count 2/Sum up new vote ==
  note: Registering votes
  Msg Header : Inport
  Enable : EnablePort
  Add : Sum
  Add1 : Sum
  Add2 : Sum
  Constant10 : Constant
  Constant11 : Constant  Value=2
  Constant12 : Constant  Value=3
  Data Store Read15 : DataStoreRead  DataStoreName=votes  DataStoreElements=votes.First_Board
  Data Store Read16 : DataStoreRead  DataStoreName=votes  DataStoreElements=votes.Second_Board
  Data Store Read17 : DataStoreRead  DataStoreName=votes  DataStoreElements=votes.Third_Board
  Data Store Write12 : DataStoreWrite  DataStoreName=votes  DataStoreElements=votes.First_Board#votes.Second_Board#votes.Third_Board
  Equal13 : RelationalOperator  Operator===  OutDataTypeStr=boolean  RndMeth=Simplest
  Equal15 : RelationalOperator  Operator===  OutDataTypeStr=boolean  RndMeth=Simplest
  Equal17 : RelationalOperator  Operator===  OutDataTypeStr=boolean  RndMeth=Simplest
  wires:
  Equal17/1 -> Add2/2
  Constant12/1 -> Equal17/1
  Add2/1 -> Data Store Write12/3
  Msg Header/1 -> Equal17/2, Equal15/2, Equal13/2
  Constant11/1 -> Equal15/1
  Data Store Read16/1 -> Add1/1
  Data Store Read15/1 -> Add/1
  Equal15/1 -> Add1/2
  Data Store Read17/1 -> Add2/1
  Constant10/1 -> Equal13/1
  Add1/1 -> Data Store Write12/2
  Add/1 -> Data Store Write12/1
  Equal13/1 -> Add/2

== system HANcoder_E407_GTSync_v4/HANcoder STM32 Target - E407-STM32 algorithm/Global Ticks Increment/CAN Management/Matrix Cycle Manager/COMP Task - Vote2 Count/Vote Count 2/Time_Difference_DEBUG ==
  RXID : Inport
  Time_Difference : Inport  Port=2
  Constant : Constant  Value=Vote1_ID
  Constant1 : Constant  Value=Vote2_ID
  Constant2 : Constant  Value=Vote3_ID
  Constant3 : Constant  Value=Sync_ID
  Data Store Read : DataStoreRead  DataStoreName=time_difference_sync
  Data Store Read1 : DataStoreRead  DataStoreName=time_difference_vote1
  Data Store Read2 : DataStoreRead  DataStoreName=time_difference_vote2
  Data Store Read3 : DataStoreRead  DataStoreName=time_difference_vote3
  Data Store Write : DataStoreWrite  DataStoreName=time_difference_sync
  Data Store Write1 : DataStoreWrite  DataStoreName=time_difference_vote1
  Data Store Write2 : DataStoreWrite  DataStoreName=time_difference_vote2
  Data Store Write3 : DataStoreWrite  DataStoreName=time_difference_vote3
  Equal{,1..3} (4 alike) : RelationalOperator  Operator===  OutDataTypeStr=boolean  RndMeth=Simplest
  Switch{,1..3} (4 alike) : Switch  Criteria=u2 > Threshold
  wires:
  Data Store Read3/1 -> Switch3/3
  Data Store Read2/1 -> Switch2/3
  Data Store Read1/1 -> Switch1/3
  Data Store Read/1 -> Switch/3
  Switch3/1 -> Data Store Write3/1  "time_difference_vote3_s2"
  Equal3/1 -> Switch3/2
  Switch2/1 -> Data Store Write2/1  "time_difference_vote2_s2"
  Switch1/1 -> Data Store Write1/1  "time_difference_vote1_s2"
  Switch/1 -> Data Store Write/1  "time_difference_sync_s2"
  Equal2/1 -> Switch2/2
  Equal1/1 -> Switch1/2
  Equal/1 -> Switch/2
  RXID/1 -> Equal/2, Equal1/2, Equal2/2, Equal3/2
  Constant2/1 -> Equal3/1
  Constant1/1 -> Equal2/1
  Constant/1 -> Equal1/1
  Constant3/1 -> Equal/1
  Time_Difference/1 -> Switch3/1, Switch2/1, Switch1/1, Switch/1

== system HANcoder_E407_GTSync_v4/HANcoder STM32 Target - E407-STM32 algorithm/Global Ticks Increment/CAN Management/Matrix Cycle Manager/COMP Task - Vote3 Count/Vote Count 3/Extra_Time ==
  Local_Time_RX : Inport
  RX_Update_Delay : Inport  Port=2
  Constant : Constant  Value=COM_Phase  OutDataTypeStr=uint16
  Minus : Sum  Inputs=++-
  Out1 : Outport  OutDataTypeStr=uint16
  wires:
  Local_Time_RX/1 -> Minus/1
  Minus/1 -> Out1/1
  RX_Update_Delay/1 -> Minus/2
  Constant/1 -> Minus/3

== system HANcoder_E407_GTSync_v4/HANcoder STM32 Target - E407-STM32 algorithm/Global Ticks Increment/CAN Management/Matrix Cycle Manager/COMP Task - Vote3 Count/Vote Count 3/Sum up new vote ==
  note: Registering votes
  Msg Header : Inport
  Enable : EnablePort
  Add : Sum
  Add1 : Sum
  Add2 : Sum
  Constant10 : Constant
  Constant11 : Constant  Value=2
  Constant12 : Constant  Value=3
  Data Store Read15 : DataStoreRead  DataStoreName=votes  DataStoreElements=votes.First_Board
  Data Store Read16 : DataStoreRead  DataStoreName=votes  DataStoreElements=votes.Second_Board
  Data Store Read17 : DataStoreRead  DataStoreName=votes  DataStoreElements=votes.Third_Board
  Data Store Write12 : DataStoreWrite  DataStoreName=votes  DataStoreElements=votes.First_Board#votes.Second_Board#votes.Third_Board
  Equal13 : RelationalOperator  Operator===  OutDataTypeStr=boolean  RndMeth=Simplest
  Equal15 : RelationalOperator  Operator===  OutDataTypeStr=boolean  RndMeth=Simplest
  Equal17 : RelationalOperator  Operator===  OutDataTypeStr=boolean  RndMeth=Simplest
  wires:
  Equal17/1 -> Add2/2
  Constant12/1 -> Equal17/1
  Add2/1 -> Data Store Write12/3
  Msg Header/1 -> Equal17/2, Equal15/2, Equal13/2
  Constant11/1 -> Equal15/1
  Data Store Read16/1 -> Add1/1
  Data Store Read15/1 -> Add/1
  Equal15/1 -> Add1/2
  Data Store Read17/1 -> Add2/1
  Constant10/1 -> Equal13/1
  Add1/1 -> Data Store Write12/2
  Add/1 -> Data Store Write12/1
  Equal13/1 -> Add/2

== system HANcoder_E407_GTSync_v4/HANcoder STM32 Target - E407-STM32 algorithm/Global Ticks Increment/CAN Management/Matrix Cycle Manager/COMP Task - Vote3 Count/Vote Count 3/Time_Difference_DEBUG ==
  RXID : Inport
  Time_Difference : Inport  Port=2
  Constant : Constant  Value=Vote1_ID
  Constant1 : Constant  Value=Vote2_ID
  Constant2 : Constant  Value=Vote3_ID
  Constant3 : Constant  Value=Sync_ID
  Data Store Read : DataStoreRead  DataStoreName=time_difference_sync
  Data Store Read1 : DataStoreRead  DataStoreName=time_difference_vote1
  Data Store Read2 : DataStoreRead  DataStoreName=time_difference_vote2
  Data Store Read3 : DataStoreRead  DataStoreName=time_difference_vote3
  Data Store Write : DataStoreWrite  DataStoreName=time_difference_sync
  Data Store Write1 : DataStoreWrite  DataStoreName=time_difference_vote1
  Data Store Write2 : DataStoreWrite  DataStoreName=time_difference_vote2
  Data Store Write3 : DataStoreWrite  DataStoreName=time_difference_vote3
  Equal{,1..3} (4 alike) : RelationalOperator  Operator===  OutDataTypeStr=boolean  RndMeth=Simplest
  Switch{,1..3} (4 alike) : Switch  Criteria=u2 > Threshold
  wires:
  Time_Difference/1 -> Switch/1, Switch1/1, Switch2/1, Switch3/1
  Constant3/1 -> Equal/1
  Constant/1 -> Equal1/1
  Constant1/1 -> Equal2/1
  Constant2/1 -> Equal3/1
  RXID/1 -> Equal3/2, Equal2/2, Equal1/2, Equal/2
  Equal/1 -> Switch/2
  Equal1/1 -> Switch1/2
  Equal2/1 -> Switch2/2
  Switch/1 -> Data Store Write/1  "time_difference_sync_s3"
  Switch1/1 -> Data Store Write1/1  "time_difference_vote1_s3"
  Switch2/1 -> Data Store Write2/1  "time_difference_vote2_s3"
  Equal3/1 -> Switch3/2
  Switch3/1 -> Data Store Write3/1  "time_difference_vote3_s3"
  Data Store Read/1 -> Switch/3
  Data Store Read1/1 -> Switch1/3
  Data Store Read2/1 -> Switch2/3
  Data Store Read3/1 -> Switch3/3

== system HANcoder_E407_GTSync_v4/HANcoder STM32 Target - E407-STM32 algorithm/Global Ticks Increment/CAN Recieve/RxID_CAN/Sync_ID_CAN/CAN receive/Enabled Subsystem ==
  In1 : Inport
  In2 : Inport  Port=2
  In3 : Inport  Port=3
  In4 : Inport  Port=4
  In5 : Inport  Port=5
  In6 : Inport  Port=6
  In7 : Inport  Port=7
  In8 : Inport  Port=8
  Enable : EnablePort
  Out1 : Outport
  Out2 : Outport  Port=2
  Out3 : Outport  Port=3
  Out4 : Outport  Port=4
  Out5 : Outport  Port=5
  Out6 : Outport  Port=6
  Out7 : Outport  Port=7
  Out8 : Outport  Port=8
  wires:
  In8/1 -> Out8/1
  In7/1 -> Out7/1
  In6/1 -> Out6/1
  In5/1 -> Out5/1
  In4/1 -> Out4/1
  In3/1 -> Out3/1
  In2/1 -> Out2/1
  In1/1 -> Out1/1

== system HANcoder_E407_GTSync_v4/HANcoder STM32 Target - E407-STM32 algorithm/Global Ticks Increment/CAN Recieve/RxID_CAN/Vote1_ID_CAN/CAN receive/Enabled Subsystem ==
  In1 : Inport
  In2 : Inport  Port=2
  In3 : Inport  Port=3
  In4 : Inport  Port=4
  In5 : Inport  Port=5
  In6 : Inport  Port=6
  In7 : Inport  Port=7
  In8 : Inport  Port=8
  Enable : EnablePort
  Out1 : Outport
  Out2 : Outport  Port=2
  Out3 : Outport  Port=3
  Out4 : Outport  Port=4
  Out5 : Outport  Port=5
  Out6 : Outport  Port=6
  Out7 : Outport  Port=7
  Out8 : Outport  Port=8
  wires:
  In1/1 -> Out1/1
  In2/1 -> Out2/1
  In3/1 -> Out3/1
  In4/1 -> Out4/1
  In5/1 -> Out5/1
  In6/1 -> Out6/1
  In7/1 -> Out7/1
  In8/1 -> Out8/1

== system HANcoder_E407_GTSync_v4/HANcoder STM32 Target - E407-STM32 algorithm/Global Ticks Increment/CAN Recieve/RxID_CAN/Vote2_ID_CAN/CAN receive/Enabled Subsystem ==
  In1 : Inport
  In2 : Inport  Port=2
  In3 : Inport  Port=3
  In4 : Inport  Port=4
  In5 : Inport  Port=5
  In6 : Inport  Port=6
  In7 : Inport  Port=7
  In8 : Inport  Port=8
  Enable : EnablePort
  Out1 : Outport
  Out2 : Outport  Port=2
  Out3 : Outport  Port=3
  Out4 : Outport  Port=4
  Out5 : Outport  Port=5
  Out6 : Outport  Port=6
  Out7 : Outport  Port=7
  Out8 : Outport  Port=8
  wires:
  In8/1 -> Out8/1
  In7/1 -> Out7/1
  In6/1 -> Out6/1
  In5/1 -> Out5/1
  In4/1 -> Out4/1
  In3/1 -> Out3/1
  In2/1 -> Out2/1
  In1/1 -> Out1/1

== system HANcoder_E407_GTSync_v4/HANcoder STM32 Target - E407-STM32 algorithm/Global Ticks Increment/CAN Recieve/RxID_CAN/Vote3_ID_CAN/CAN receive/Enabled Subsystem ==
  In1 : Inport
  In2 : Inport  Port=2
  In3 : Inport  Port=3
  In4 : Inport  Port=4
  In5 : Inport  Port=5
  In6 : Inport  Port=6
  In7 : Inport  Port=7
  In8 : Inport  Port=8
  Enable : EnablePort
  Out1 : Outport
  Out2 : Outport  Port=2
  Out3 : Outport  Port=3
  Out4 : Outport  Port=4
  Out5 : Outport  Port=5
  Out6 : Outport  Port=6
  Out7 : Outport  Port=7
  Out8 : Outport  Port=8
  wires:
  In1/1 -> Out1/1
  In2/1 -> Out2/1
  In3/1 -> Out3/1
  In4/1 -> Out4/1
  In5/1 -> Out5/1
  In6/1 -> Out6/1
  In7/1 -> Out7/1
  In8/1 -> Out8/1

== system HANcoder_E407_GTSync_v4/HANcoder STM32 Target - E407-STM32 algorithm/Global Ticks Increment/CAN Management/Matrix Cycle Manager/COMP Task - Update LT/Local Time Update/Process Time Difference/Check_Wrap_up ==
  In1 : Inport
  GreaterThan : RelationalOperator  Operator=>  OutDataTypeStr=boolean  RndMeth=Simplest
  Minus : Sum  Inputs=+-
  Switch : Switch  Criteria=u2 > Threshold
  Wrap-up_Threshold : Constant  Value=wrap_up_threshold
  Wrap-up_Threshold1 : Constant  Value=basic_cycle_duration
  Out1 : Outport
  wires:
  In1/1 -> Minus/1, Switch/3, GreaterThan/1
  Wrap-up_Threshold/1 -> GreaterThan/2
  GreaterThan/1 -> Switch/2
  Switch/1 -> Out1/1
  Minus/1 -> Switch/1
  Wrap-up_Threshold1/1 -> Minus/2

== system HANcoder_E407_GTSync_v4/HANcoder STM32 Target - E407-STM32 algorithm/Global Ticks Increment/CAN Management/Matrix Cycle Manager/COMP Task - Update LT/Local Time Update/Process Time Difference/Check_Wrap_up1 ==
  In1 : Inport
  GreaterThan : RelationalOperator  Operator=>  OutDataTypeStr=boolean  RndMeth=Simplest
  Minus : Sum  Inputs=+-
  Switch : Switch  Criteria=u2 > Threshold
  Wrap-up_Threshold : Constant  Value=wrap_up_threshold
  Wrap-up_Threshold1 : Constant  Value=basic_cycle_duration
  Out1 : Outport
  wires:
  Wrap-up_Threshold1/1 -> Minus/2
  Minus/1 -> Switch/1
  Switch/1 -> Out1/1
  GreaterThan/1 -> Switch/2
  Wrap-up_Threshold/1 -> GreaterThan/2
  In1/1 -> GreaterThan/1, Switch/3, Minus/1

== system HANcoder_E407_GTSync_v4/HANcoder STM32 Target - E407-STM32 algorithm/Global Ticks Increment/CAN Management/Matrix Cycle Manager/COMP Task - Update LT1/Local Time Update/Process Time Difference/Check_Wrap_up ==
  In1 : Inport
  GreaterThan : RelationalOperator  Operator=>  OutDataTypeStr=boolean  RndMeth=Simplest
  Minus : Sum  Inputs=+-
  Switch : Switch  Criteria=u2 > Threshold
  Wrap-up_Threshold : Constant  Value=wrap_up_threshold
  Wrap-up_Threshold1 : Constant  Value=basic_cycle_duration
  Out1 : Outport
  wires:
  Wrap-up_Threshold1/1 -> Minus/2
  Minus/1 -> Switch/1
  Switch/1 -> Out1/1
  GreaterThan/1 -> Switch/2
  Wrap-up_Threshold/1 -> GreaterThan/2
  In1/1 -> GreaterThan/1, Switch/3, Minus/1
